simulink model "raw_diagram"  (R2020b)
settings: Solver=VariableStepAuto  StartTime=0.0  StopTime=10.0  RelTol=1e-3
values from neighbouring files (symbols this model uses):
  i = 60    [Untitled.m]    (also in driver.m = 196; maks.m = 546)
  J = 1.3    [Untitled.m]    (also in driver.m = 0.39; maks.m = 0.15)
  k = 0.1375    [Untitled.m]    (also in driver.m = 0.14; maks.m = 0.004; old_hw.m = 1; research.m = 1)
undefined symbols (not defined in the file or in its folder): Jp, Km, ku, L, nu, r
settings Model: Creator=morro  LastModifiedBy=morro

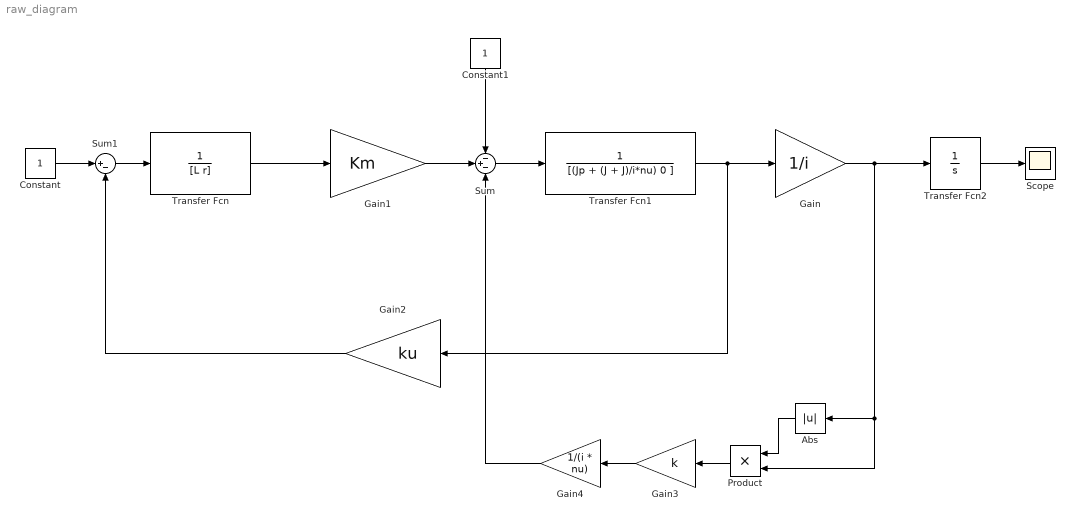
== system raw_diagram ==
  Abs : Abs
  Constant : Constant
  Constant1 : Constant
  Gain : Gain  Gain=1/i
  Gain1 : Gain  Gain=Km
  Gain2 : Gain  Gain=ku
  Gain3 : Gain  Gain=k
  Gain4 : Gain  Gain=1/(i * nu)
  Product : Product
  Scope : Scope
  Sum : Sum  Inputs=-+-
  Sum1 : Sum  Inputs=|+-
  Transfer Fcn : TransferFcn  Denominator=[L r]
  Transfer Fcn1 : TransferFcn  Denominator=[(Jp + (J + J)/i*nu) 0 ]
  Transfer Fcn2 : TransferFcn  Denominator=[1 0]
  wires:
  Transfer Fcn2/1 -> Scope/1
  Transfer Fcn/1 -> Gain1/1
  Gain1/1 -> Sum/2
  Constant/1 -> Sum1/1
  Sum/1 -> Transfer Fcn1/1
  Constant1/1 -> Sum/1
  Sum1/1 -> Transfer Fcn/1
  Abs/1 -> Product/1
  Gain3/1 -> Gain4/1
  Gain2/1 -> Sum1/2
  Transfer Fcn1/1 -> Gain2/1, Gain/1
  Gain4/1 -> Sum/3
  Gain/1 -> Abs/1, Product/2, Transfer Fcn2/1
  Product/1 -> Gain3/1
